simulink model "Linear_Gust"  (R2020b)
settings: Solver=VariableStepAuto  StartTime=0.0  StopTime=100  RelTol=1e-3
values from neighbouring files (symbols this model uses):
  g = 9.81    [Angular_gust.mat]    (also in Linear_gust.mat; Real_Values.m; Trial_Script.m; TryingNewAeroCoeffs.m)
  m = 941.102    [Angular_gust.mat]    (also in Linear_gust.mat; Real_Values.m; Trial_Script.m = 645; TryingNewAeroCoeffs.m)
  r_cgCatia = [0.0401998 0.00180957 -0.293434]    [Angular_gust.mat]    (also in Linear_gust.mat; Real_Values.m = TcgCatia*r_cgCatia; Trial_Script.m = [2; 0; 0]; TryingNewAeroCoeffs.m = TcgCatia*r_cgCatia)
  r_trajectory = [0 0 0]    [Angular_gust.mat]    (also in Linear_gust.mat; Real_Values.m = [0;0;0]; Trial_Script.m = [0;0;0]; TryingNewAeroCoeffs.m = [0;0;0])
  rho = 1.225    [Angular_gust.mat]    (also in Linear_gust.mat; Real_Values.m; Trial_Script.m; TryingNewAeroCoeffs.m)
  T = 10.5    [Angular_gust.mat]    (also in Linear_gust.mat; Real_Values.m; Trial_Script.m; TryingNewAeroCoeffs.m)
  TcgCatia = [1  0  0; 0  -1  0; 0  0  -1]    [Angular_gust.mat]    (also in Linear_gust.mat; Real_Values.m = [1 0 0; Trial_Script.m = [1 0 0; TryingNewAeroCoeffs.m = [1 0 0)
  time_delay = 0.01    [Angular_gust.mat]    (also in Linear_gust.mat; Real_Values.m = 0.1; Trial_Script.m = 0.1; TryingNewAeroCoeffs.m)
  ZI_Cx = [4.10002314469 4.10486511138 4.10970707807 4.11454904475 4.11939101144 4.12423297813 4.12907494481 4.1339169115 4.13875887819 4.14360084487 4.14844281156 4.15328477825 ... (65341 elements, 361x181)]    [Angular_gust.mat]    (also in Linear_gust.mat; Real_Values.m = model_Cx(XI_Cx, YI_Cx); Trial_Script.m = model_Cx(XI_Cx, YI_Cx); TryingNewAeroCoeffs.m = model_Cx(XI_Cx, YI_Cx))
  ZI_Cy = [5.10662222372 5.15407485934 5.20152749496 5.24898013059 5.29643276621 5.34388540184 5.39133803746 5.43879067308 5.48624330871 5.53369594433 5.58114857996 5.62860121558 ... (65341 elements, 361x181)]    [Angular_gust.mat]    (also in Linear_gust.mat; Real_Values.m = model_Cy(XI_Cy, YI_Cy); Trial_Script.m = model_Cy(XI_Cy, YI_Cy); TryingNewAeroCoeffs.m = model_Cy(XI_Cy, YI_Cy))
  ZI_Cz = [-10.5947720774 -10.6317912004 -10.6688103235 -10.7058294465 -10.7428485695 -10.7798676926 -10.8168868156 -10.8539059387 -10.8909250617 -10.9279441847 -10.9649633078 -11.0019824308 ... (65341 elements, 361x181)]    [Angular_gust.mat]    (also in Linear_gust.mat; Real_Values.m = model_Cz(XI_Cz, YI_Cz); Trial_Script.m = model_Cz(XI_Cz, YI_Cz); TryingNewAeroCoeffs.m = model_Cz(XI_Cz, YI_Cz))
  ZI_p = [6.05111971338 6.06712776392 6.08313581446 6.099143865 6.11515191553 6.13115996607 6.14716801661 6.16317606715 6.17918411769 6.19519216823 6.21120021877 6.22720826931 ... (65341 elements, 361x181)]    [Angular_gust.mat]    (also in Linear_gust.mat; Real_Values.m = model_p(XI_p, YI_p); Trial_Script.m = model_p(XI_p, YI_p); TryingNewAeroCoeffs.m = model_p(XI_p, YI_p))
  ZI_q = [0.071083987219 0.054175962948 0.0372679386771 0.0203599144061 0.00345189013513 -0.0134561341358 -0.0303641584068 -0.0472721826778 -0.0641802069487 -0.0810882312197 -0.0979962554907 -0.114904279762 ... (65341 elements, 361x181)]    [Angular_gust.mat]    (also in Linear_gust.mat; Real_Values.m = model_q(XI_q, YI_q); Trial_Script.m = model_q(XI_q, YI_q); TryingNewAeroCoeffs.m = model_q(XI_q, YI_q))
  ZI_r = [-1.8762921931 -1.88364224017 -1.89099228723 -1.8983423343 -1.90569238136 -1.91304242842 -1.92039247549 -1.92774252255 -1.93509256961 -1.94244261668 -1.94979266374 -1.95714271081 ... (65341 elements, 361x181)]    [Angular_gust.mat]    (also in Linear_gust.mat; Real_Values.m = model_r(XI_r, YI_r); Trial_Script.m = model_r(XI_r, YI_r); TryingNewAeroCoeffs.m = model_r(XI_r, YI_r))
libraries: pid_lib x3, sharedutil x1
settings Model: Creator=Jonathan van Zyl  LastModifiedBy=Jonathan van Zyl

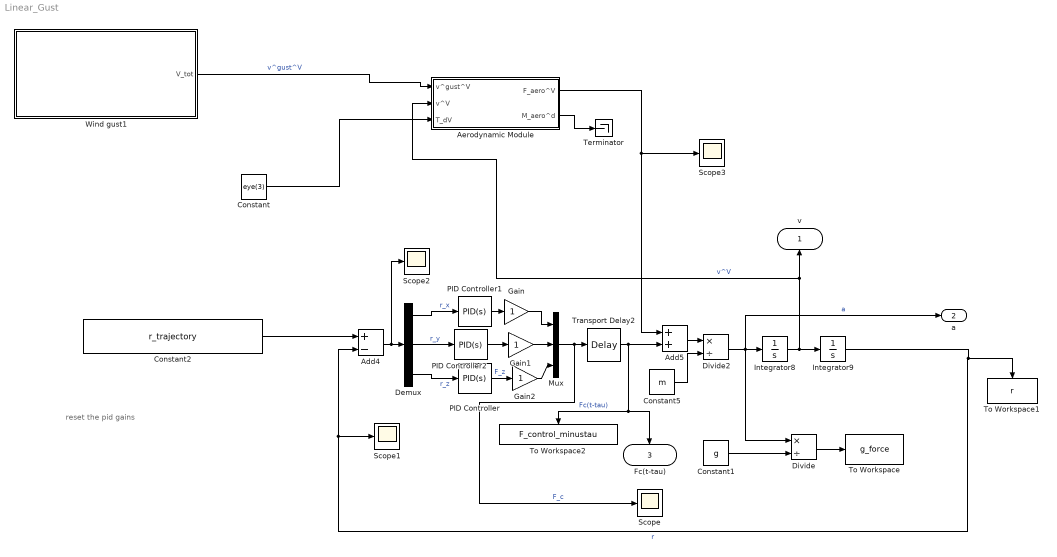
== system Linear_Gust ==
  note: reset the pid gains
  Add4 : Sum  Inputs=+-
  Add5 : Sum
  Aerodynamic Module : Subsystem
  Constant : Constant  Value=eye(3)
  Constant1 : Constant  Value=g
  Constant2 : Constant  Value=r_trajectory
  Constant5 : Constant  Value=m
  Demux : Demux  Outputs=3
  Divide : Product  Inputs=*/
  Divide2 : Product  Inputs=*/
  Gain : Gain
  Gain1 : Gain
  Gain2 : Gain
  Integrator8 : Integrator
  Integrator9 : Integrator
  Mux : Mux  Inputs=3
  PID Controller : pid_lib/PID Controller  Controller=PID  Form=Parallel  TimeDomain=Continuous-time  UseExternalTs=off  SampleTime=-1  IntegratorMethod=Forward Euler  FilterMethod=Forward Euler  ControllerParametersSource=internal  P=160.734193661502  I=6.85755125615993  D=923.025793270617  UseFilter=on  N=10.4897155810233  TunerSelectOption=Transfer Function Based (PID Tuner App)  InitialConditionSource=internal  InitialConditionForIntegrator=0  InitialConditionForFilter=0  DifferentiatorICPrevScaledInput=0  ExternalReset=none  TrackingMode=off  Kt=1  LimitOutput=off  SatLimitsSource=internal  UpperSaturationLimit=inf  LowerSaturationLimit=-inf  LinearizeAsGain=on  AntiWindupMode=none  Kb=1  POutMin=[]  POutMax=[]  IOutMin=[]  IOutMax=[]  DOutMin=[]  DOutMax=[]  NOutMin=[]  NOutMax=[]  SumOutMin=[]  SumOutMax=[]  SaturationOutMin=[]  SaturationOutMax=[]  PParamMin=[]  PParamMax=[]  IParamMin=[]  IParamMax=[]  DParamMin=[]  DParamMax=[]  NParamMin=[]  NParamMax=[]  KbParamMin=[]  KbParamMax=[]  KtParamMin=[]  KtParamMax=[]  KbOutMin=[]  KbOutMax=[]  KtOutMin=[]  KtOutMax=[]  IntegratorOutMin=[]  IntegratorOutMax=[]  FilterOutMin=[]  FilterOutMax=[]  SumI1OutMin=[]  SumI1OutMax=[]  SumI2OutMin=[]  SumI2OutMax=[]  SumI3OutMin=[]  SumI3OutMax=[]  SumI4OutMin=[]  SumI4OutMax=[]  SumDOutMin=[]  SumDOutMax=[]  DifferentiatorOutMin=[]  DifferentiatorOutMax=[]  FilterDiffOutCoefMin=[]  FilterDiffOutCoefMax=[]  ReciprocalOutMin=[]  ReciprocalOutMax=[]  SumDenOutMin=[]  SumDenOutMax=[]  SumNumOutMin=[]  SumNumOutMax=[]  DivideOutMin=[]  DivideOutMax=[]  UdiffTsProdOutMin=[]  UdiffTsProdOutMax=[]  NTsProdOutMin=[]  NTsProdOutMax=[]  UintegralTsProdOutMin=[]  UintegralTsProdOutMax=[]  UngainTsProdOutMin=[]  UngainTsProdOutMax=[]  IntegratorContinuousStateAttributes=''  IntegratorStateMustResolveToSignalObject=off  IntegratorRTWStateStorageClass=Auto  FilterContinuousStateAttributes=''  FilterStateMustResolveToSignalObject=off  FilterRTWStateStorageClass=Auto  ParallelPVariant=InternalParameters  IdealPVariant=Disabled  IVariant=InternalParameters  DVariant=InternalParameters  IntegratorVariant=Continuous  SatVariant=Disabled  AWVariant=Passthrough  PCopyVariant=Disabled  TRVariant=Disabled  FdbkBlocksVariant=Forward  IdealPFdbkVariant=Disabled  SatFdbkVariant=Disabled  DerivativeFilterVariant=ContFilter  NVariant=InternalParameters  NCopyVariant=Disabled  FilterICVariant=InternalICsFilter  IntegratorICVariant=InternalICs  ExternalResetVariant=Disabled  TRSumVariant=Passthrough  SumFdbkVariant=Disabled  SumVariant=Sum_PID  TsampFilterVariant=InternalTs  TsampNgainVariant=Passthrough  TsampIntegralVariant=Passthrough  ExternalSaturationOutDataTypeStr=Inherit: Same as second input
  PID Controller1 : pid_lib/PID Controller  Controller=PID  Form=Parallel  TimeDomain=Continuous-time  UseExternalTs=off  SampleTime=-1  IntegratorMethod=Forward Euler  FilterMethod=Forward Euler  ControllerParametersSource=internal  P=160.734193661502  I=6.85755125615993  D=923.025793270617  UseFilter=on  N=10.4897155810233  TunerSelectOption=Transfer Function Based (PID Tuner App)  InitialConditionSource=internal  InitialConditionForIntegrator=0  InitialConditionForFilter=0  DifferentiatorICPrevScaledInput=0  ExternalReset=none  TrackingMode=off  Kt=1  LimitOutput=off  SatLimitsSource=internal  UpperSaturationLimit=inf  LowerSaturationLimit=-inf  LinearizeAsGain=on  AntiWindupMode=none  Kb=1  POutMin=[]  POutMax=[]  IOutMin=[]  IOutMax=[]  DOutMin=[]  DOutMax=[]  NOutMin=[]  NOutMax=[]  SumOutMin=[]  SumOutMax=[]  SaturationOutMin=[]  SaturationOutMax=[]  PParamMin=[]  PParamMax=[]  IParamMin=[]  IParamMax=[]  DParamMin=[]  DParamMax=[]  NParamMin=[]  NParamMax=[]  KbParamMin=[]  KbParamMax=[]  KtParamMin=[]  KtParamMax=[]  KbOutMin=[]  KbOutMax=[]  KtOutMin=[]  KtOutMax=[]  IntegratorOutMin=[]  IntegratorOutMax=[]  FilterOutMin=[]  FilterOutMax=[]  SumI1OutMin=[]  SumI1OutMax=[]  SumI2OutMin=[]  SumI2OutMax=[]  SumI3OutMin=[]  SumI3OutMax=[]  SumI4OutMin=[]  SumI4OutMax=[]  SumDOutMin=[]  SumDOutMax=[]  DifferentiatorOutMin=[]  DifferentiatorOutMax=[]  FilterDiffOutCoefMin=[]  FilterDiffOutCoefMax=[]  ReciprocalOutMin=[]  ReciprocalOutMax=[]  SumDenOutMin=[]  SumDenOutMax=[]  SumNumOutMin=[]  SumNumOutMax=[]  DivideOutMin=[]  DivideOutMax=[]  UdiffTsProdOutMin=[]  UdiffTsProdOutMax=[]  NTsProdOutMin=[]  NTsProdOutMax=[]  UintegralTsProdOutMin=[]  UintegralTsProdOutMax=[]  UngainTsProdOutMin=[]  UngainTsProdOutMax=[]  IntegratorContinuousStateAttributes=''  IntegratorStateMustResolveToSignalObject=off  IntegratorRTWStateStorageClass=Auto  FilterContinuousStateAttributes=''  FilterStateMustResolveToSignalObject=off  FilterRTWStateStorageClass=Auto  ParallelPVariant=InternalParameters  IdealPVariant=Disabled  IVariant=InternalParameters  DVariant=InternalParameters  IntegratorVariant=Continuous  SatVariant=Disabled  AWVariant=Passthrough  PCopyVariant=Disabled  TRVariant=Disabled  FdbkBlocksVariant=Forward  IdealPFdbkVariant=Disabled  SatFdbkVariant=Disabled  DerivativeFilterVariant=ContFilter  NVariant=InternalParameters  NCopyVariant=Disabled  FilterICVariant=InternalICsFilter  IntegratorICVariant=InternalICs  ExternalResetVariant=Disabled  TRSumVariant=Passthrough  SumFdbkVariant=Disabled  SumVariant=Sum_PID  TsampFilterVariant=InternalTs  TsampNgainVariant=Passthrough  TsampIntegralVariant=Passthrough  ExternalSaturationOutDataTypeStr=Inherit: Same as second input
  PID Controller2 : pid_lib/PID Controller  Controller=PID  Form=Parallel  TimeDomain=Continuous-time  UseExternalTs=off  SampleTime=-1  IntegratorMethod=Forward Euler  FilterMethod=Forward Euler  ControllerParametersSource=internal  P=160.734193661502  I=6.85755125615993  D=923.025793270617  UseFilter=on  N=10.4897155810233  TunerSelectOption=Transfer Function Based (PID Tuner App)  InitialConditionSource=internal  InitialConditionForIntegrator=0  InitialConditionForFilter=0  DifferentiatorICPrevScaledInput=0  ExternalReset=none  TrackingMode=off  Kt=1  LimitOutput=off  SatLimitsSource=internal  UpperSaturationLimit=inf  LowerSaturationLimit=-inf  LinearizeAsGain=on  AntiWindupMode=none  Kb=1  POutMin=[]  POutMax=[]  IOutMin=[]  IOutMax=[]  DOutMin=[]  DOutMax=[]  NOutMin=[]  NOutMax=[]  SumOutMin=[]  SumOutMax=[]  SaturationOutMin=[]  SaturationOutMax=[]  PParamMin=[]  PParamMax=[]  IParamMin=[]  IParamMax=[]  DParamMin=[]  DParamMax=[]  NParamMin=[]  NParamMax=[]  KbParamMin=[]  KbParamMax=[]  KtParamMin=[]  KtParamMax=[]  KbOutMin=[]  KbOutMax=[]  KtOutMin=[]  KtOutMax=[]  IntegratorOutMin=[]  IntegratorOutMax=[]  FilterOutMin=[]  FilterOutMax=[]  SumI1OutMin=[]  SumI1OutMax=[]  SumI2OutMin=[]  SumI2OutMax=[]  SumI3OutMin=[]  SumI3OutMax=[]  SumI4OutMin=[]  SumI4OutMax=[]  SumDOutMin=[]  SumDOutMax=[]  DifferentiatorOutMin=[]  DifferentiatorOutMax=[]  FilterDiffOutCoefMin=[]  FilterDiffOutCoefMax=[]  ReciprocalOutMin=[]  ReciprocalOutMax=[]  SumDenOutMin=[]  SumDenOutMax=[]  SumNumOutMin=[]  SumNumOutMax=[]  DivideOutMin=[]  DivideOutMax=[]  UdiffTsProdOutMin=[]  UdiffTsProdOutMax=[]  NTsProdOutMin=[]  NTsProdOutMax=[]  UintegralTsProdOutMin=[]  UintegralTsProdOutMax=[]  UngainTsProdOutMin=[]  UngainTsProdOutMax=[]  IntegratorContinuousStateAttributes=''  IntegratorStateMustResolveToSignalObject=off  IntegratorRTWStateStorageClass=Auto  FilterContinuousStateAttributes=''  FilterStateMustResolveToSignalObject=off  FilterRTWStateStorageClass=Auto  ParallelPVariant=InternalParameters  IdealPVariant=Disabled  IVariant=InternalParameters  DVariant=InternalParameters  IntegratorVariant=Continuous  SatVariant=Disabled  AWVariant=Passthrough  PCopyVariant=Disabled  TRVariant=Disabled  FdbkBlocksVariant=Forward  IdealPFdbkVariant=Disabled  SatFdbkVariant=Disabled  DerivativeFilterVariant=ContFilter  NVariant=InternalParameters  NCopyVariant=Disabled  FilterICVariant=InternalICsFilter  IntegratorICVariant=InternalICs  ExternalResetVariant=Disabled  TRSumVariant=Passthrough  SumFdbkVariant=Disabled  SumVariant=Sum_PID  TsampFilterVariant=InternalTs  TsampNgainVariant=Passthrough  TsampIntegralVariant=Passthrough  ExternalSaturationOutDataTypeStr=Inherit: Same as second input
  Scope{,1..3} (4 alike) : Scope
  Terminator : Terminator
  To Workspace : ToWorkspace  VariableName=g_force  SaveFormat=Timeseries  SampleTime=-1
      settings: Save2DSignal=2-D array (concatenate along first dimension)
  To Workspace1 : ToWorkspace  VariableName=r  SaveFormat=Timeseries  SampleTime=-1
  To Workspace2 : ToWorkspace  VariableName=F_control_minustau  SaveFormat=Timeseries  SampleTime=-1
  Transport Delay2 : TransportDelay  DelayTime=time_delay  TransDelayFeedthrough=on
  Wind gust1 : Subsystem
  v : Outport
  a : Outport  Port=2
  Fc(t-tau) : Outport  Port=3
  wires:
  Integrator8/1 -> Aerodynamic Module/2(v^V), v/1, Integrator9/1  "v^V"
  Integrator9/1 -> Scope1/1, Add4/2, To Workspace1/1  "r"
  Gain1/1 -> Mux/2
  Transport Delay2/1 -> Add5/2, Fc(t-tau)/1, To Workspace2/1  "Fc(t-tau)"
  Demux/2 -> PID Controller2/1  "r_y"
  PID Controller1/1 -> Gain/1
  Add5/1 -> Divide2/1
  Gain2/1 -> Mux/3
  PID Controller/1 -> Gain2/1  "F_z"
  Divide2/1 -> a/1, Integrator8/1, Divide/1  "a"
  Constant1/1 -> Divide/2
  PID Controller2/1 -> Gain1/1
  Divide/1 -> To Workspace/1
  Constant2/1 -> Add4/1
  Add4/1 -> Scope2/1, Demux/1
  Constant5/1 -> Divide2/2
  Demux/3 -> PID Controller/1  "r_z"
  Mux/1 -> Scope/1, Transport Delay2/1  "F_c"
  Gain/1 -> Mux/1
  Demux/1 -> PID Controller1/1  "r_x"
  Constant/1 -> Aerodynamic Module/3(T_dV)
  Aerodynamic Module/2(M_aero^d) -> Terminator/1
  Wind gust1/1(V_tot) -> Aerodynamic Module/1(v^gust^V)  "v^gust^V"
  Aerodynamic Module/1(F_aero^V) -> Scope3/1, Add5/1

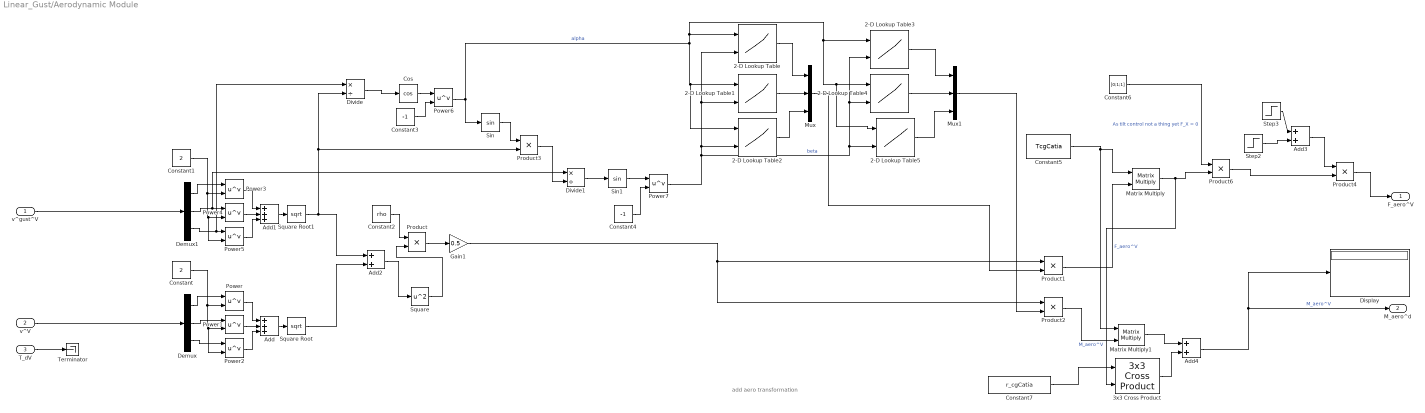
== system Linear_Gust/Aerodynamic Module ==
  note: add aero transformation
  v^gust^V : Inport
  v^V : Inport  Port=2
  T_dV : Inport  Port=3
  2-D Lookup Table : Lookup_n-D  BreakpointsForDimension1=[-180:1:180]  BreakpointsForDimension2=[-180:1:180]  Table=ZI_Cx  InternalRulePriority=Speed  RndMeth=Simplest  InputSameDT=on
      settings: InputPortMap=u0,u1
  2-D Lookup Table1 : Lookup_n-D  BreakpointsForDimension1=[-180:1:180]  BreakpointsForDimension2=[-180:1:180]  Table=ZI_Cy  InternalRulePriority=Speed  RndMeth=Simplest  InputSameDT=on
      settings: InputPortMap=u0,u1
  2-D Lookup Table2 : Lookup_n-D  BreakpointsForDimension1=[-180:1:180]  BreakpointsForDimension2=[-180:1:180]  Table=ZI_Cz  InternalRulePriority=Speed  RndMeth=Simplest  InputSameDT=on
      settings: InputPortMap=u0,u1
  2-D Lookup Table3 : Lookup_n-D  BreakpointsForDimension1=[-180:1:180]  BreakpointsForDimension2=[-180:1:180]  Table=ZI_p  InternalRulePriority=Speed  RndMeth=Simplest  InputSameDT=on
      settings: InputPortMap=u0,u1
  2-D Lookup Table4 : Lookup_n-D  BreakpointsForDimension1=[-180:1:180]  BreakpointsForDimension2=[-180:1:180]  Table=ZI_q  InternalRulePriority=Speed  RndMeth=Simplest  InputSameDT=on
      settings: InputPortMap=u0,u1
  2-D Lookup Table5 : Lookup_n-D  BreakpointsForDimension1=[-180:1:180]  BreakpointsForDimension2=[-180:1:180]  Table=ZI_r  InternalRulePriority=Speed  RndMeth=Simplest  InputSameDT=on
      settings: InputPortMap=u0,u1
  3x3 Cross Product : sharedutil/3x3 Cross Product  aMode=aMode
      settings: SourceProductBaseCode=AE,PW,MT,UV,VE,VP
  Add : Sum  Inputs=+++
  Add1 : Sum  Inputs=+++
  Add2 : Sum
  Add3 : Sum
  Add4 : Sum
  Constant : Constant  Value=2
  Constant1 : Constant  Value=2
  Constant2 : Constant  Value=rho
  Constant3 : Constant  Value=-1
  Constant4 : Constant  Value=-1
  Constant5 : Constant  Value=TcgCatia
  Constant6 : Constant  Value=[0;1;1]
  Constant7 : Constant  Value=r_cgCatia
  Cos : Trigonometry  Operator=cos
  Demux : Demux  Outputs=3
  Demux1 : Demux  Outputs=3
  Display : Display
  Divide : Product  Inputs=*/
  Divide1 : Product  Inputs=*/
  Gain1 : Gain  Gain=0.5
  Matrix Multiply : Product  Multiplication=Matrix(*)
  Matrix Multiply1 : Product  Multiplication=Matrix(*)
  Mux : Mux  Inputs=3
  Mux1 : Mux  Inputs=3
  Power{,1..7} (8 alike) : Math  Operator=pow  SaturateOnIntegerOverflow=on
  Product{,1..4,6} (6 alike) : Product
  Sin : Trigonometry
  Sin1 : Trigonometry
  Square : Math  Operator=square  SaturateOnIntegerOverflow=on
  Square Root : Sqrt  SaturateOnIntegerOverflow=on
  Square Root1 : Sqrt  SaturateOnIntegerOverflow=on
  Step2 : Step  Time=0  SampleTime=0
  Step3 : Step  Time=10.5  After=-1  SampleTime=0
  Terminator : Terminator
  F_aero^V : Outport
  M_aero^d : Outport  Port=2
  wires:
  Constant1/1 -> Power5/2, Power4/2, Power3/2
  Product1/1 -> Matrix Multiply/2  "F_aero^V"
  Square Root/1 -> Add2/2
  Power6/1 -> Sin/1, 2-D Lookup Table/1, 2-D Lookup Table5/1, 2-D Lookup Table4/1, 2-D Lookup Table3/1, 2-D Lookup Table2/1, 2-D Lookup Table1/1  "alpha"
  Power1/1 -> Add/2
  2-D Lookup Table5/1 -> Mux1/3
  Constant/1 -> Power2/2, Power1/2, Power/2
  Divide/1 -> Cos/1
  Demux/1 -> Power/1
  Power5/1 -> Add1/3
  2-D Lookup Table/1 -> Mux/1
  Divide1/1 -> Sin1/1
  Demux1/1 -> Power3/1
  Add2/1 -> Square/1
  Add4/1 -> Display/1, M_aero^d/1  "M_aero^V"
  Demux/3 -> Power2/1
  Constant4/1 -> Power7/2
  2-D Lookup Table4/1 -> Mux1/2
  Gain1/1 -> Product2/1, Product1/1
  Constant3/1 -> Power6/2
  Power7/1 -> 2-D Lookup Table/2, 2-D Lookup Table1/2, 2-D Lookup Table2/2, 2-D Lookup Table3/2, 2-D Lookup Table4/2, 2-D Lookup Table5/2  "beta"
  Cos/1 -> Power6/1
  Demux1/3 -> Divide/1, Power5/1
  Product/1 -> Gain1/1
  Sin1/1 -> Power7/1
  Power2/1 -> Add/3
  Sin/1 -> Product3/1
  Mux1/1 -> Product2/2
  Demux1/2 -> Divide1/1, Power4/1
  Power4/1 -> Add1/2
  Add/1 -> Square Root/1
  Power/1 -> Add/1
  Square Root1/1 -> Product3/2, Divide/2, Add2/1
  v^gust^V/1 -> Demux1/1
  2-D Lookup Table3/1 -> Mux1/1
  2-D Lookup Table1/1 -> Mux/2
  Power3/1 -> Add1/1
  Mux/1 -> Product1/2
  Product3/1 -> Divide1/2
  2-D Lookup Table2/1 -> Mux/3
  Add1/1 -> Square Root1/1
  Constant2/1 -> Product/1
  Demux/2 -> Power1/1
  v^V/1 -> Demux/1
  Square/1 -> Product/2
  Constant6/1 -> Product6/1  "As tilt control not a thing yet F_X = 0"
  Product6/1 -> Product4/2
  T_dV/1 -> Terminator/1
  Constant5/1 -> Matrix Multiply1/1, Matrix Multiply/1
  Matrix Multiply/1 -> 3x3 Cross Product/2, Product6/2
  Constant7/1 -> 3x3 Cross Product/1
  Matrix Multiply1/1 -> Add4/1
  3x3 Cross Product/1 -> Add4/2
  Product2/1 -> Matrix Multiply1/2  "M_aero^V"
  Step2/1 -> Add3/2
  Step3/1 -> Add3/1
  Add3/1 -> Product4/1
  Product4/1 -> F_aero^V/1

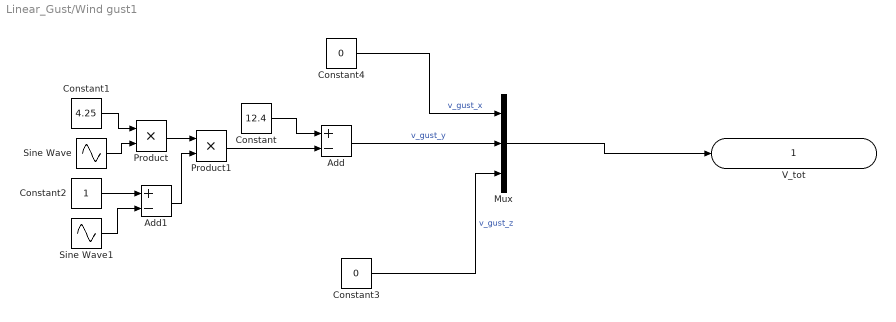
== system Linear_Gust/Wind gust1 ==
  Add : Sum  Inputs=+-
  Add1 : Sum  Inputs=+-
  Constant : Constant  Value=12.4
  Constant1 : Constant  Value=4.25
  Constant2 : Constant
  Constant3 : Constant  Value=0
  Constant4 : Constant  Value=0  VectorParams1D=off
  Mux : Mux  Inputs=3
  Product : Product
  Product1 : Product
  Sine Wave : Sin  Frequency=3*pi/T  SampleTime=0
  Sine Wave1 : Sin  Frequency=2*pi/T  Phase=pi/2  SampleTime=0
  V_tot : Outport
  wires:
  Constant/1 -> Add/1
  Constant1/1 -> Product/1
  Sine Wave/1 -> Product/2
  Constant2/1 -> Add1/1
  Sine Wave1/1 -> Add1/2
  Product/1 -> Product1/1
  Add1/1 -> Product1/2
  Product1/1 -> Add/2
  Add/1 -> Mux/2  "v_gust_y"
  Constant3/1 -> Mux/3  "v_gust_z"
  Constant4/1 -> Mux/1  "v_gust_x"
  Mux/1 -> V_tot/1
